simulink model "Exercise632"  (R2017a)
settings: Solver=VariableStepAuto  StartTime=0.0  StopTime=2  RelTol=1e-3  EnableMultiTasking=on
undefined symbols (not defined in the file): Dens, f, J, ke, kt, L, Nums, R
settings Model: Creator=Ramiro  LastModifiedBy=JakobLab
settings OptimizationCC: LifeSpan=inf
settings DebuggingCC: SFUnexpectedBacktrackingDiag=warning  SFNoUnconditionalDefaultTransitionDiag=warning  SFExecutionAtInitializationDiag=none
settings GRTTargetCC: TargetLangStandard=C89/C90 (ANSI)  GeneratePreprocessorConditionals=Disable all
settings ConfigComp: CovMetricSettings=dw  CovHtmlReporting=on  CovSaveCumulativeToWorkspaceVar=on  CovSaveSingleToWorkspaceVar=on  CovExternalEMLEnable=off

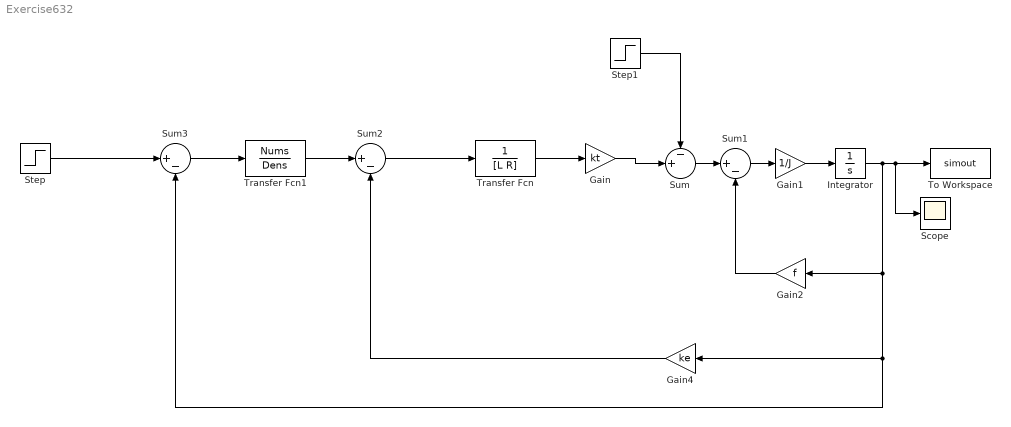
== system Exercise632 ==
  Gain : Gain  Gain=kt
  Gain1 : Gain  Gain=1/J
  Gain2 : Gain  Gain=f
  Gain4 : Gain  Gain=ke
  Integrator : Integrator
  Scope : Scope
  Step : Step  Time=0  After=5  SampleTime=0
  Step1 : Step  Time=0.5  After=0.001  SampleTime=0
  Sum : Sum  Inputs=-+|
  Sum1 : Sum  Inputs=|+-
  Sum2 : Sum  Inputs=|+-
  Sum3 : Sum  Inputs=|+-
  To Workspace : ToWorkspace  VariableName=simout  SaveFormat=Structure With Time  SampleTime=-1
  Transfer Fcn : TransferFcn  Denominator=[L R]
  Transfer Fcn1 : TransferFcn  Numerator=Nums  Denominator=Dens
  wires:
  Gain/1 -> Sum/2
  Step1/1 -> Sum/1
  Sum/1 -> Sum1/1
  Sum1/1 -> Gain1/1
  Gain2/1 -> Sum1/2
  Transfer Fcn/1 -> Gain/1
  Sum2/1 -> Transfer Fcn/1
  Gain1/1 -> Integrator/1
  Gain4/1 -> Sum2/2
  Integrator/1 -> To Workspace/1, Scope/1, Gain4/1, Sum3/2, Gain2/1
  Step/1 -> Sum3/1
  Sum3/1 -> Transfer Fcn1/1
  Transfer Fcn1/1 -> Sum2/1
